simulink model "Exemplu_figura10"  (R2016a)
settings: Solver=VariableStepAuto  StartTime=0.0  StopTime=10.0  RelTol=1e-3
undefined symbols (not defined in the file): entity, f, m, n
settings Model: Creator=Cristina  LastModifiedBy=Cristina

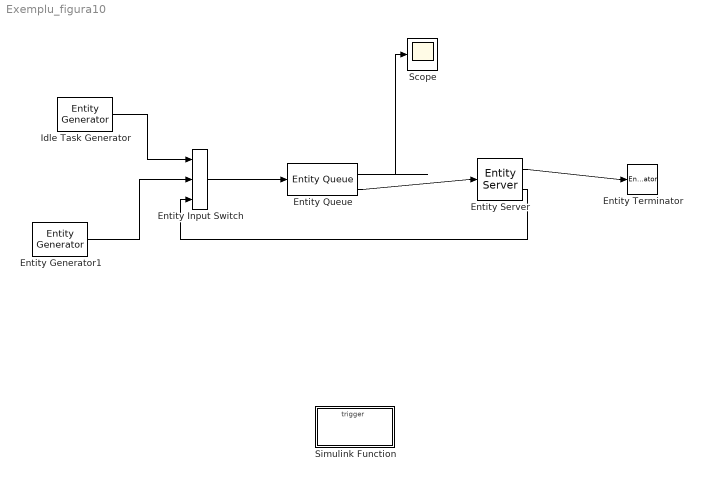
== system Exemplu_figura10 ==
  Entity Input Switch : EntityInputSwitch  InputPortMessageModes=m,m,m  OutputPortMessageModes=m  NumberInputPorts=3
      settings: InputPortMap=u1,u2,u3
  Entity Generator1 : EntityGenerator  OutputPortMessageModes=m  TimeSource=MATLAB action  IntergenerationTimeAction=|  AttributeName=Priority|ServiceTime  AttributeInitialValue=1|1  EntityType=Structured  EntityTypeName=Entity
      | persistent init
      | if (isempty(init))
      |      rng (123);
      |      init = true;
      | end
      | dt = 1.6 * rand + 0.4;
  Entity Queue : EntityQueue  InputPortMessageModes=m  OutputPortMessageModes=n,m  QueueType=Priority  PrioritySource=Priority  ExitAction=f(entity.Priority);  NumberEntitiesInBlock=on
      settings: OutputPortMap=o1,o5
  Entity Server : EntityServer  InputPortMessageModes=m  OutputPortMessageModes=m,m  Capacity=1  PermitPreemptionBasedOnAttribute=on  SortingAttributeName=Priority
      settings: OutputPortMap=o9,o10
  Entity Terminator : EntityTerminator  InputPortMessageModes=m
  Idle Task Generator : EntityGenerator  OutputPortMessageModes=m  Period=inf  AttributeName=Priority|ServiceTime  AttributeInitialValue=100|inf  EntityType=Structured  EntityTypeName=Entity
  Scope : Scope
  Simulink Function : Subsystem  TreatAsAtomicUnit=on
  wires:
  Entity Input Switch/1 -> Entity Queue/1
  Entity Queue/2 -> Entity Server/1
  Entity Server/1 -> Entity Terminator/1
  Idle Task Generator/1 -> Entity Input Switch/1
  Entity Generator1/1 -> Entity Input Switch/2
  Entity Server/2 -> Entity Input Switch/3
  Entity Queue/1 -> Scope/1

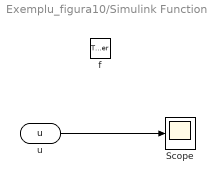
== system Exemplu_figura10/Simulink Function ==
  f : TriggerPort  TriggerType=function-call  IsSimulinkFunction=on  FunctionName=f  VariantControl=Variant
  Scope : Scope
  u : ArgIn  DisableCoverage=on  ArgumentName=u
  wires:
  u/1 -> Scope/1
